simulink model "EPD629_WilliamsJ_AS07_Simulink"  (R2021b)
settings: Solver=VariableStepAuto  StartTime=0.0  StopTime=30  MaxStep=0.01  RelTol=1e-3
values from neighbouring files (symbols this model uses):
  AirGasConstant_kJpkgK = 0.287    [EPD629_WilliamsJ_AS07.m]
  AirToFuelEquivalenceRatio_frac = 1    [EPD629_WilliamsJ_AS07.m]
  AmbientPressure_kPa = 98    [EPD629_WilliamsJ_AS07.m]
  BaseSparkAdvanceData_deg = min(MBTSparkAdvanceData_deg,BorderlineSparkAdvData_deg)    [EPD629_WilliamsJ_AS07.m]
  CrankAngleIVCToTDC_deg = 170    [EPD629_WilliamsJ_AS07.m]
  CylinderAirMassBreakpoints_mg = 0:25:400    [EPD629_WilliamsJ_AS07.m]
  DelayFuelInjectionToIVC_rev = 0.75    [EPD629_WilliamsJ_AS07.m]
  DelayFuelInjectionToIVCEst_rev = 0.75    [EPD629_WilliamsJ_AS07.m]
  DelayIVCToOxygenSensor_rev = 7    [EPD629_WilliamsJ_AS07.m]
  DischargeCoefficient_frac = 0.7    [EPD629_WilliamsJ_AS07.m]
  EngineDisplacement_L = 2.77    [EPD629_WilliamsJ_AS07.m]
  EngineInertia_kgm2 = 0.2    [EPD629_WilliamsJ_AS07.m]
  EngineMotoringFrictionData_Nm = Beta_0 + Beta_2*Omega_e.^2    [EPD629_WilliamsJ_AS07.m]
  EngineSpeedBreakpoints_rpm = 400:200:5000    [EPD629_WilliamsJ_AS07.m]
  FuelControlIntegralGain = 2e-5    (= 2e-05)    [EPD629_WilliamsJ_AS07.m]
  FuelControlProportionalGain = 5e-6    (= 5e-06)    [EPD629_WilliamsJ_AS07.m]
  FuelInjEvapTimeConstant_s = 0.8    [EPD629_WilliamsJ_AS07.m]
  FuelInjEvapTimeConstantEst_s = 0.8    [EPD629_WilliamsJ_AS07.m]
  FuelInjImpactFactor_frac = 0.3    [EPD629_WilliamsJ_AS07.m]
  FuelInjImpactFactorEst_frac = 0.3    [EPD629_WilliamsJ_AS07.m]
  FuelLowerHeatingValue_kJpkg = 44000    [EPD629_WilliamsJ_AS07.m]
  InletAirTemperature_K = 298    [EPD629_WilliamsJ_AS07.m]
  IntakeManifoldVolume_L = 5.8    [EPD629_WilliamsJ_AS07.m]
  ManifoldAirTemperature_K = 340    [EPD629_WilliamsJ_AS07.m]
  ManifoldPressureBreakpoints_kPa = 5:5:100    [EPD629_WilliamsJ_AS07.m]
  NumberOfCylinders = 6    [EPD629_WilliamsJ_AS07.m]
  OxygenSensorLambdaBP_frac = [0 0.9 0.92 0.94 0.96 0.985 0.999 1.001 1.015 1.04 1.06 1.08 1.1 2]    [EPD629_WilliamsJ_AS07.m]
  OxygenSensorSwitchSetpoint_mV = 450    [EPD629_WilliamsJ_AS07.m]
  OxygenSensorVoltageData_mV = [800 800 794 788 775 750 700 200 150 125 112 106 100 100]    [EPD629_WilliamsJ_AS07.m]
  SparkTorqFactorData_frac = 1 - (SparkTorqFactorRetFromMBTBP_deg.^2) /      (SparkTorqFactorRetFromMBTBP_deg(end)^2)    [EPD629_WilliamsJ_AS07.m]
  SparkTorqFactorRetFromMBTBP_deg = 0:5:45    [EPD629_WilliamsJ_AS07.m]
  StoichiometricAFR_frac = 14.7    [EPD629_WilliamsJ_AS07.m]
  ThermodynamicEfficiencyData_frac = Eta_0 + Eta_1*Omega_e + Eta_2*Omega_e.^2    [EPD629_WilliamsJ_AS07.m]
  ThrottleAreaBreakpoints_pct = ThrottleAreaData_pct    [EPD629_WilliamsJ_AS07.m]
  ThrottleAreaData_pct = 100 * ThrottleArea_mm2 / WideOpenThrottleArea_mm2    [EPD629_WilliamsJ_AS07.m]
  ThrottleFlowFunctionData_frac = PR.^(1/RatioOfSpecificHeats_frac) .*      sqrt( 2 * RatioOfSpecificHeats_frac / (RatioOfSpecificHeats_frac - 1) .*      (1 - PR.^((RatioOfSpecificHeats_frac - 1) / RatioOfSpecificHeats_frac)) )    [EPD629_WilliamsJ_AS07.m]
  ThrottleMassFlowCorrIntGain = 10    [EPD629_WilliamsJ_AS07.m]
  ThrottlePositionBreakpoints_pct = 0:100    [EPD629_WilliamsJ_AS07.m]
  ThrottlePositionData_pct = ThrottlePositionBreakpoints_pct    [EPD629_WilliamsJ_AS07.m]
  ThrottlePressureRatioBreakpoints_frac = 0:0.01:1    [EPD629_WilliamsJ_AS07.m]
  VECorrectionFactorIntGain = 0.02    [EPD629_WilliamsJ_AS07.m]
  WideOpenThrottleArea_mm2 = ThrottleArea_mm2(end)    [EPD629_WilliamsJ_AS07.m]
undefined symbols (not defined in the file or in its folder): MBTSparkAdvanceData_deg, VolumetricEfficiencyData_frac
libraries: simulink x1
settings Model: Creator=Justin  LastModifiedBy=jwilli42

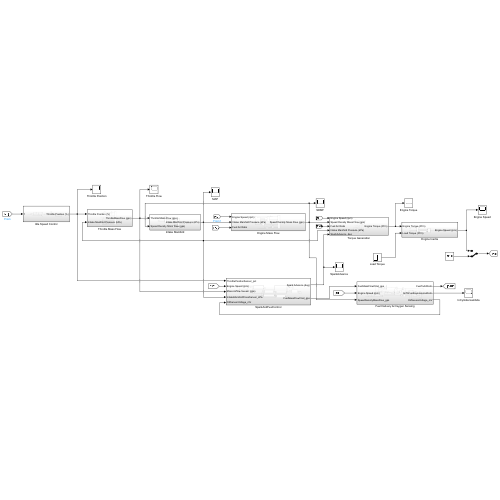
[thumbnail: Simulink's stored preview of the top-level diagram]
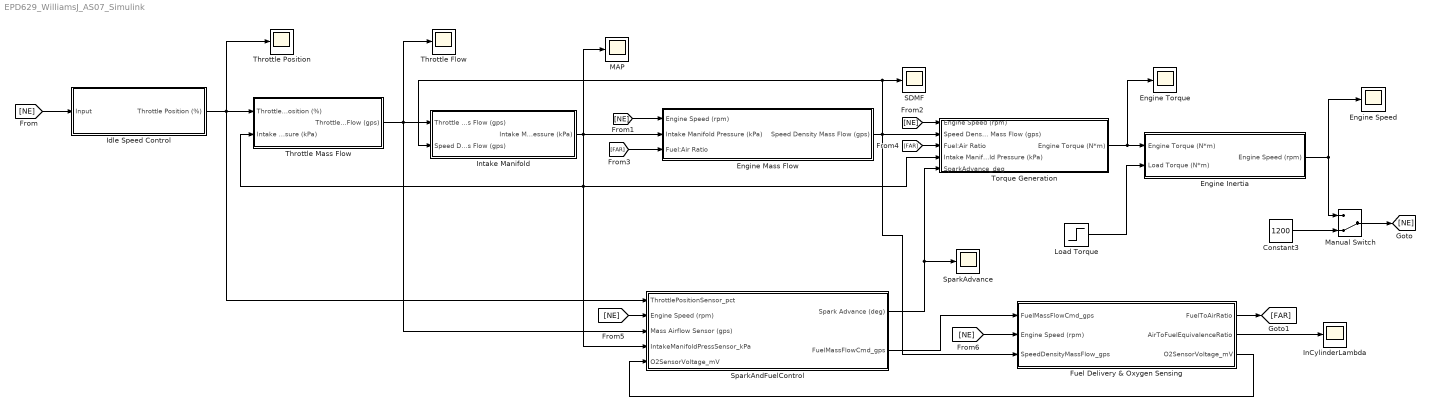
== system EPD629_WilliamsJ_AS07_Simulink ==
  Constant3 : Constant  Value=1200
  Engine Inertia : Subsystem
  Engine Mass Flow : Subsystem
  Engine Speed : Scope
  Engine Torque : Scope
  Fuel Delivery & Oxygen Sensing : Subsystem
  Idle Speed Control : Subsystem
  InCylinderLambda : Scope
  Intake Manifold : Subsystem
  Load Torque : Step  Time=5  Before=15  After=25  SampleTime=0
  MAP : Scope
  Manual Switch : ManualSwitch  CurrentSetting=0
  SDMF : Scope
  SparkAdvance : Scope
  SparkAndFuelControl : Subsystem
  Throttle Flow : Scope
  Throttle Mass Flow : Subsystem
  Throttle Position : Scope
  Torque Generation : Subsystem
  wires:
  Load Torque/1 -> Engine Inertia/2(Load Torque (N*m))
  Idle Speed Control/1(Throttle Position (%)) -> Throttle Mass Flow/1(Throttle Position (%)), SparkAndFuelControl/1(ThrottlePositionSensor_pct), Throttle Position/1
  Intake Manifold/1(Intake Manifold Pressure (kPa)) -> Torque Generation/4(Intake Manifold Pressure (kPa)), SparkAndFuelControl/4(IntakeManifoldPressSensor_kPa), Throttle Mass Flow/2(Intake Manifold Pressure (kPa)), MAP/1, Engine Mass Flow/2(Intake Manifold Pressure (kPa))
  Engine Mass Flow/1(Speed Density Mass Flow (gps)) -> Fuel Delivery & Oxygen Sensing/3(SpeedDensityMassFlow_gps), Torque Generation/2(Speed Density Mass Flow (gps)), SDMF/1, Intake Manifold/2(Speed Density Mass Flow (gps))
  Torque Generation/1(Engine Torque (N*m)) -> Engine Torque/1, Engine Inertia/1(Engine Torque (N*m))
  Engine Inertia/1(Engine Speed (rpm)) -> Engine Speed/1, Manual Switch/1
  [NE] -> Idle Speed Control/1(Input)
  [NE] -> Engine Mass Flow/1(Engine Speed (rpm))
  [NE] -> Torque Generation/1(Engine Speed (rpm))
  [FAR] -> Torque Generation/3(Fuel:Air Ratio)
  [FAR] -> Engine Mass Flow/3(Fuel:Air Ratio)
  Manual Switch/1 -> [NE]
  Constant3/1 -> Manual Switch/2
  SparkAndFuelControl/1(Spark Advance (deg)) -> SparkAdvance/1, Torque Generation/5(SparkAdvance_deg)
  Fuel Delivery & Oxygen Sensing/2(AirToFuelEquivalenceRatio) -> InCylinderLambda/1
  Fuel Delivery & Oxygen Sensing/1(FuelToAirRatio) -> [FAR]
  Fuel Delivery & Oxygen Sensing/3(O2SensorVoltage_mV) -> SparkAndFuelControl/5(O2SensorVoltage_mV)
  [NE] -> SparkAndFuelControl/2(Engine Speed (rpm))
  Throttle Mass Flow/1(ThrottleMassFlow (gps)) -> SparkAndFuelControl/3(Mass Airflow Sensor (gps)), Intake Manifold/1(Throttle Mass Flow (gps)), Throttle Flow/1
  [NE] -> Fuel Delivery & Oxygen Sensing/2(Engine Speed (rpm))
  SparkAndFuelControl/2(FuelMassFlowCmd_gps) -> Fuel Delivery & Oxygen Sensing/1(FuelMassFlowCmd_gps)

== system EPD629_WilliamsJ_AS07_Simulink/Engine Inertia ==
  Engine Torque (N*m) : Inport
  Load Torque (N*m) : Inport  Port=2
  Constant : Constant  Value=EngineInertia_kgm2
  Divide : Product  Inputs=*/
  Engine Speed : Integrator  InitialCondition=600  LimitOutput=on  UpperSaturationLimit=5000  LowerSaturationLimit=0
  Subtract : Sum  Inputs=+-
  rad/s^2 to rpm/s : Gain  Gain=30/pi
  Engine Speed (rpm) : Outport
  wires:
  Engine Torque (N*m)/1 -> Subtract/1
  Load Torque (N*m)/1 -> Subtract/2
  Subtract/1 -> Divide/1
  Constant/1 -> Divide/2
  Divide/1 -> rad/s^2 to rpm/s/1
  rad/s^2 to rpm/s/1 -> Engine Speed/1
  Engine Speed/1 -> Engine Speed (rpm)/1

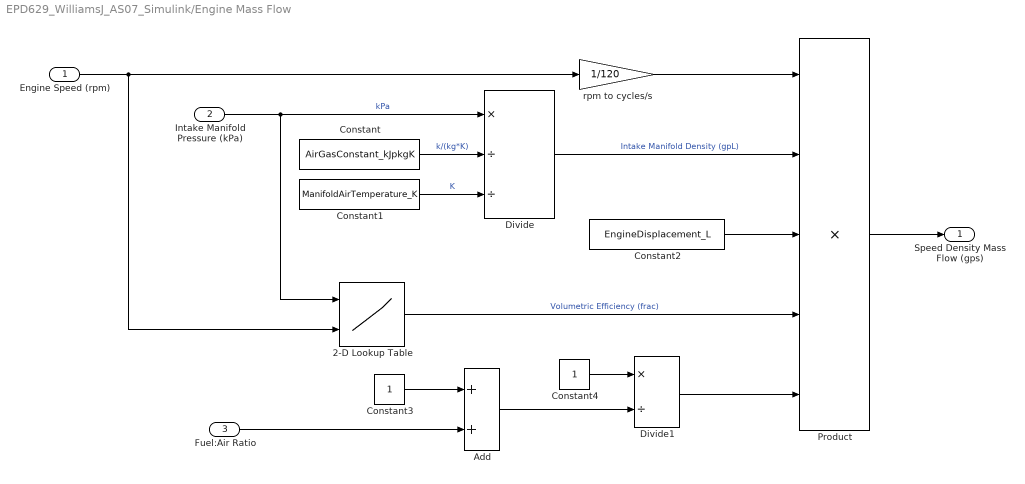
== system EPD629_WilliamsJ_AS07_Simulink/Engine Mass Flow ==
  Engine Speed (rpm) : Inport
  Intake Manifold Pressure (kPa) : Inport  Port=2
  Fuel:Air Ratio : Inport  Port=3
  2-D Lookup Table : Lookup_n-D  BreakpointsForDimension1=ManifoldPressureBreakpoints_kPa  BreakpointsForDimension2=EngineSpeedBreakpoints_rpm  Table=VolumetricEfficiencyData_frac  ExtrapMethod=Clip  UseLastTableValue=on  InternalRulePriority=Speed  RndMeth=Simplest  InputSameDT=on
      settings: InputPortMap=u0,u1
  Add : Sum
  Constant : Constant  Value=AirGasConstant_kJpkgK
  Constant1 : Constant  Value=ManifoldAirTemperature_K
  Constant2 : Constant  Value=EngineDisplacement_L
  Constant3 : Constant
  Constant4 : Constant
  Divide : Product  Inputs=*//
  Divide1 : Product  Inputs=*/
  Product : Product  Inputs=5
  rpm to cycles/s : Gain  Gain=1/120
  Speed Density Mass Flow (gps) : Outport
  wires:
  Engine Speed (rpm)/1 -> rpm to cycles/s/1, 2-D Lookup Table/2
  Intake Manifold Pressure (kPa)/1 -> Divide/1, 2-D Lookup Table/1  "kPa"
  Constant/1 -> Divide/2  "k/(kg*K)"
  Constant1/1 -> Divide/3  "K"
  rpm to cycles/s/1 -> Product/1
  Divide/1 -> Product/2  "Intake Manifold Density (gpL)"
  Constant2/1 -> Product/3
  2-D Lookup Table/1 -> Product/4  "Volumetric Efficiency (frac)"
  Constant3/1 -> Add/1
  Fuel:Air Ratio/1 -> Add/2
  Constant4/1 -> Divide1/1
  Add/1 -> Divide1/2
  Divide1/1 -> Product/5
  Product/1 -> Speed Density Mass Flow (gps)/1

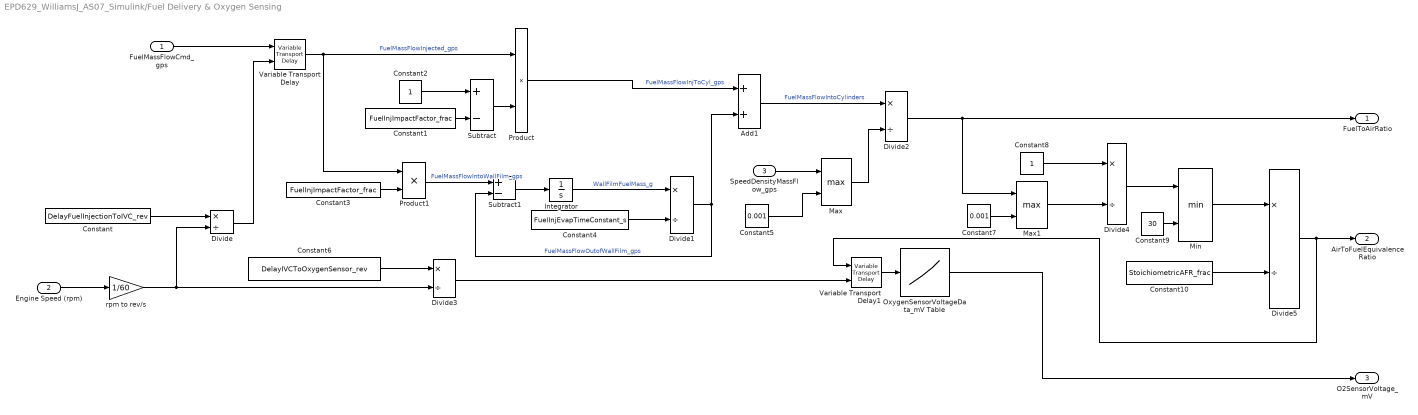
== system EPD629_WilliamsJ_AS07_Simulink/Fuel Delivery & Oxygen Sensing ==
  FuelMassFlowCmd_gps : Inport
  Engine Speed (rpm) : Inport  Port=2
  SpeedDensityMassFlow_gps : Inport  Port=3
  Add1 : Sum
  Constant : Constant  Value=DelayFuelInjectionToIVC_rev
  Constant1 : Constant  Value=FuelInjImpactFactor_frac
  Constant10 : Constant  Value=StoichiometricAFR_frac
  Constant2 : Constant
  Constant3 : Constant  Value=FuelInjImpactFactor_frac
  Constant4 : Constant  Value=FuelInjEvapTimeConstant_s
  Constant5 : Constant  Value=0.001
  Constant6 : Constant  Value=DelayIVCToOxygenSensor_rev
  Constant7 : Constant  Value=0.001
  Constant8 : Constant
  Constant9 : Constant  Value=30
  Divide{,1..5} (6 alike) : Product  Inputs=*/
  Integrator : Integrator  InitialCondition=.015  LimitOutput=on  LowerSaturationLimit=0
  Max : MinMax  Function=max  Inputs=2
  Max1 : MinMax  Function=max  Inputs=2
  Min : MinMax  Inputs=2
  OxygenSensorVoltageData_mV Table : Lookup_n-D  NumberOfTableDimensions=1  BreakpointsForDimension1=OxygenSensorLambdaBP_frac  Table=OxygenSensorVoltageData_mV  ExtrapMethod=Clip  UseLastTableValue=on  InternalRulePriority=Speed  RndMeth=Simplest  InputSameDT=on
  Product : Product
  Product1 : Product
  Subtract : Sum  Inputs=+-
  Subtract1 : Sum  Inputs=+-
  Variable Transport Delay : VariableTransportDelay  VariableDelayType=Variable transport delay  MaximumDelay=10  InitialOutput=.165  MaximumPoints=10000
  Variable Transport Delay1 : VariableTransportDelay  VariableDelayType=Variable transport delay  MaximumDelay=10  InitialOutput=1
  rpm to rev/s : Gain  Gain=1/60
  FuelToAirRatio : Outport
  AirToFuelEquivalenceRatio : Outport  Port=2
  O2SensorVoltage_mV : Outport  Port=3
  wires:
  FuelMassFlowCmd_gps/1 -> Variable Transport Delay/1
  Engine Speed (rpm)/1 -> rpm to rev/s/1
  Constant/1 -> Divide/1
  rpm to rev/s/1 -> Divide/2, Divide3/2
  Divide/1 -> Variable Transport Delay/2
  Constant1/1 -> Subtract/2
  Constant2/1 -> Subtract/1
  Subtract/1 -> Product/2
  Variable Transport Delay/1 -> Product1/1, Product/1  "FuelMassFlowInjected_gps"
  Product/1 -> Add1/1  "FuelMassFlowInjToCyl_gps"
  Constant3/1 -> Product1/2
  Product1/1 -> Subtract1/1  "FuelMassFlowIntoWallFilm_gps"
  Subtract1/1 -> Integrator/1
  Integrator/1 -> Divide1/1  "WallFilmFuelMass_g"
  Constant4/1 -> Divide1/2
  Divide1/1 -> Add1/2, Subtract1/2  "FuelMassFlowOutofWallFilm_gps"
  Add1/1 -> Divide2/1  "FuelMassFlowIntoCylinders"
  SpeedDensityMassFlow_gps/1 -> Max/1
  Constant5/1 -> Max/2
  Max/1 -> Divide2/2
  Constant6/1 -> Divide3/1
  Divide3/1 -> Variable Transport Delay1/2
  Constant7/1 -> Max1/2
  Max1/1 -> Divide4/2
  Constant8/1 -> Divide4/1
  Divide2/1 -> FuelToAirRatio/1, Max1/1
  Divide4/1 -> Min/1
  Constant9/1 -> Min/2
  Constant10/1 -> Divide5/2
  Min/1 -> Divide5/1
  Divide5/1 -> Variable Transport Delay1/1, AirToFuelEquivalenceRatio/1
  Variable Transport Delay1/1 -> OxygenSensorVoltageData_mV Table/1
  OxygenSensorVoltageData_mV Table/1 -> O2SensorVoltage_mV/1

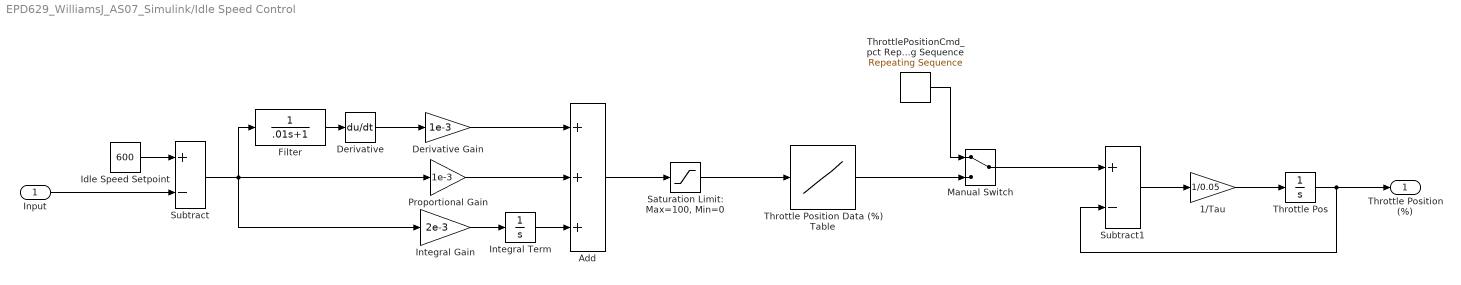
== system EPD629_WilliamsJ_AS07_Simulink/Idle Speed Control ==
  Input : Inport
  1/Tau : Gain  Gain=1/0.05
  Add : Sum  Inputs=+++
  Derivative : Derivative
  Derivative Gain : Gain  Gain=1e-3
  Filter : TransferFcn  Denominator=[.01 1]
  Idle Speed Setpoint : Constant  Value=600
  Integral Gain : Gain  Gain=2e-3
  Integral Term : Integrator  InitialCondition=0.6  LimitOutput=on  UpperSaturationLimit=100  LowerSaturationLimit=0
  Manual Switch : ManualSwitch
  Proportional Gain : Gain  Gain=1e-3
  "Saturation Limit: Max=100, Min=0" : Saturate  UpperLimit=100  LowerLimit=0
  Subtract : Sum  Inputs=+-
  Subtract1 : Sum  Inputs=+-
  Throttle Pos : Integrator  InitialCondition=1.7  LimitOutput=on  UpperSaturationLimit=100  LowerSaturationLimit=0
  Throttle Position Data (%) Table : Lookup_n-D  NumberOfTableDimensions=1  BreakpointsForDimension1=ThrottleAreaBreakpoints_pct  Table=ThrottlePositionData_pct  ExtrapMethod=Clip  UseLastTableValue=on  InternalRulePriority=Speed  RndMeth=Simplest  InputSameDT=on
  ThrottlePositionCmd_pct Repeating Sequence : simulink/Sources/Repeating Sequence  rep_seq_t=[0, 4.5, 5, 9.5, 10]  rep_seq_y=[5, 5, 15, 15, 5]
  Throttle Position (%) : Outport
  wires:
  Idle Speed Setpoint/1 -> Subtract/1
  Filter/1 -> Derivative/1
  Subtract/1 -> Integral Gain/1, Filter/1, Proportional Gain/1
  Derivative/1 -> Derivative Gain/1
  Derivative Gain/1 -> Add/1
  Proportional Gain/1 -> Add/2
  Integral Gain/1 -> Integral Term/1
  Integral Term/1 -> Add/3
  Input/1 -> Subtract/2
  Add/1 -> "Saturation Limit: Max=100, Min=0"/1
  "Saturation Limit: Max=100, Min=0"/1 -> Throttle Position Data (%) Table/1
  Throttle Position Data (%) Table/1 -> Manual Switch/2
  Subtract1/1 -> 1/Tau/1
  1/Tau/1 -> Throttle Pos/1
  Throttle Pos/1 -> Subtract1/2, Throttle Position (%)/1
  Manual Switch/1 -> Subtract1/1
  ThrottlePositionCmd_pct Repeating Sequence/1 -> Manual Switch/1

== system EPD629_WilliamsJ_AS07_Simulink/Intake Manifold ==
  Throttle Mass Flow (gps) : Inport
  Speed Density Mass Flow (gps) : Inport  Port=2
  Constant : Constant  Value=AirGasConstant_kJpkgK
  Constant1 : Constant  Value=ManifoldAirTemperature_K
  Constant2 : Constant  Value=IntakeManifoldVolume_L
  Divide : Product  Inputs=***/
  MAP (kPa) : Integrator  InitialCondition=33.5  LimitOutput=on  UpperSaturationLimit=110  LowerSaturationLimit=10
  Subtract : Sum  Inputs=+-
  Intake Manifold Pressure (kPa) : Outport
  wires:
  Throttle Mass Flow (gps)/1 -> Subtract/1
  Speed Density Mass Flow (gps)/1 -> Subtract/2
  Subtract/1 -> Divide/1  "dm/dt"
  Constant/1 -> Divide/2
  Constant1/1 -> Divide/3
  Constant2/1 -> Divide/4
  Divide/1 -> MAP (kPa)/1  "dP_m/dt"
  MAP (kPa)/1 -> Intake Manifold Pressure (kPa)/1  "P_m"

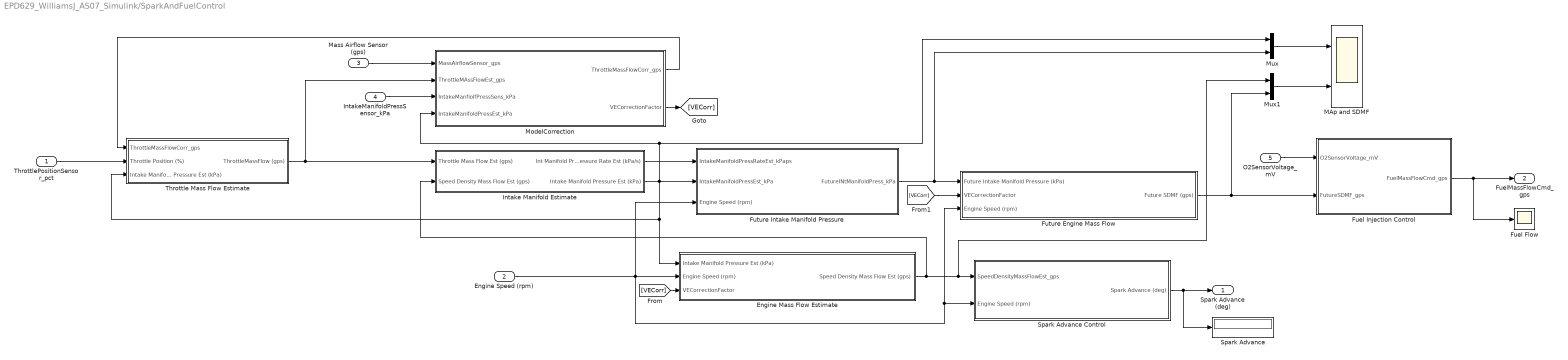
== system EPD629_WilliamsJ_AS07_Simulink/SparkAndFuelControl ==
  ThrottlePositionSensor_pct : Inport
  Engine Speed (rpm) : Inport  Port=2
  Mass Airflow Sensor (gps) : Inport  Port=3
  IntakeManifoldPressSensor_kPa : Inport  Port=4
  O2SensorVoltage_mV : Inport  Port=5
  Engine Mass Flow Estimate : Subsystem
  Fuel Flow : Scope
  "Fuel Injection Control " : Subsystem
  Future Engine Mass Flow : Subsystem
  Future Intake Manifold Pressure : Subsystem
  Intake Manifold Estimate : Subsystem
  MAp and SDMF : Scope  NumInputPorts=2
  ModelCorrection : Subsystem
  Mux : Mux  Inputs=2
  Mux1 : Mux  Inputs=2
  Spark Advance : Display
  Spark Advance Control : Subsystem
  Throttle Mass Flow Estimate : Subsystem
  Spark Advance (deg) : Outport
  FuelMassFlowCmd_gps : Outport  Port=2
  wires:
  Throttle Mass Flow Estimate/1(ThrottleMassFlow (gps)) -> Intake Manifold Estimate/1(Throttle Mass Flow Est (gps)), ModelCorrection/2(ThrottleMAssFlowEst_gps)
  ThrottlePositionSensor_pct/1 -> Throttle Mass Flow Estimate/2(Throttle Position (%))
  ModelCorrection/1(ThrottleMassFlowCorr_gps) -> Throttle Mass Flow Estimate/1(ThrottleMassFlowCorr_gps)
  Engine Speed (rpm)/1 -> Spark Advance Control/2(Engine Speed (rpm)), Future Engine Mass Flow/3(Engine Speed (rpm)), Engine Mass Flow Estimate/2(Engine Speed (rpm)), Future Intake Manifold Pressure/3(Engine Speed (rpm))
  Intake Manifold Estimate/2(Intake Manifold Pressure Est (kPa)) -> Mux/1, ModelCorrection/4(IntakeManifoldPressEst_kPa), Future Intake Manifold Pressure/2(IntakeManifoldPressEst_kPa), Throttle Mass Flow Estimate/3(Intake Manifold Pressure Est (kPa)), Engine Mass Flow Estimate/1(Intake Manifold Pressure Est (kPa))
  Intake Manifold Estimate/1(Int Manifold Pressure Rate Est (kPa/s)) -> Future Intake Manifold Pressure/1(IntakeManifoldPressRateEst_kPaps)
  Engine Mass Flow Estimate/1(Speed Density Mass Flow Est (gps)) -> Intake Manifold Estimate/2(Speed Density Mass Flow Est (gps)), Spark Advance Control/1(SpeedDensityMassFlowEst_gps), Mux1/1
  Future Intake Manifold Pressure/1(FutureINtManifoldPress_kPa) -> Mux/2, Future Engine Mass Flow/1(Future Intake Manifold Pressure (kPa))
  Future Engine Mass Flow/1(Future SDMF (gps)) -> Mux1/2, "Fuel Injection Control "/2(FutureSDMF_gps)
  Spark Advance Control/1(Spark Advance (deg)) -> Spark Advance/1, Spark Advance (deg)/1
  [VECorr] -> Engine Mass Flow Estimate/3(VECorrectionFactor)
  ModelCorrection/2(VECorrectionFactor) -> [VECorr]
  Mass Airflow Sensor (gps)/1 -> ModelCorrection/1(MassAirflowSensor_gps)
  IntakeManifoldPressSensor_kPa/1 -> ModelCorrection/3(IntakeManfiolfPressSens_kPa)
  O2SensorVoltage_mV/1 -> "Fuel Injection Control "/1(O2SensorVoltage_mV)
  "Fuel Injection Control "/1(FuelMassFlowCmd_gps) -> Fuel Flow/1, FuelMassFlowCmd_gps/1
  [VECorr] -> Future Engine Mass Flow/2(VECorrectionFactor)
  Mux/1 -> MAp and SDMF/1
  Mux1/1 -> MAp and SDMF/2

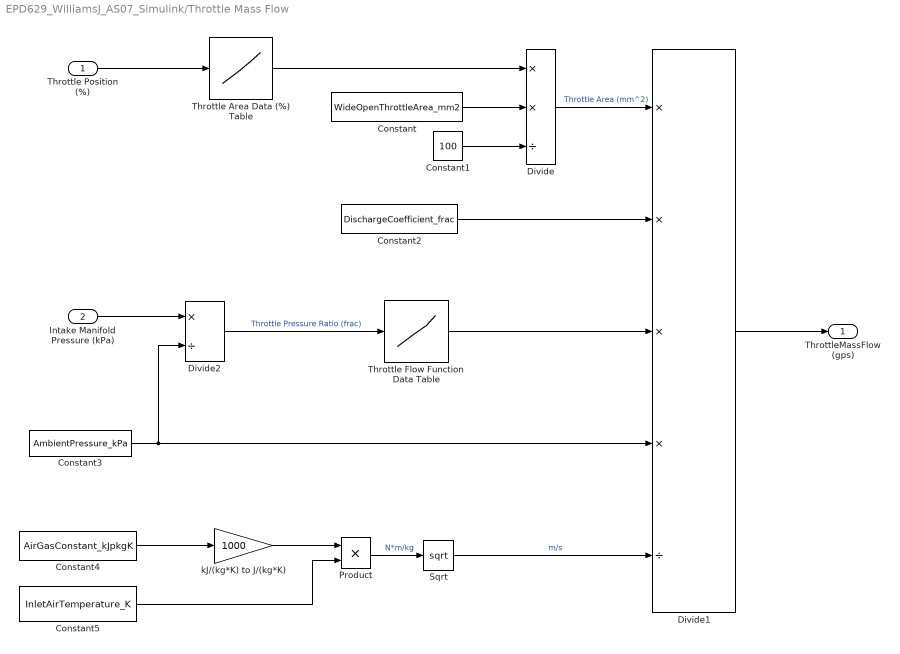
== system EPD629_WilliamsJ_AS07_Simulink/Throttle Mass Flow ==
  Throttle Position (%) : Inport
  Intake Manifold Pressure (kPa) : Inport  Port=2
  Constant : Constant  Value=WideOpenThrottleArea_mm2
  Constant1 : Constant  Value=100
  Constant2 : Constant  Value=DischargeCoefficient_frac
  Constant3 : Constant  Value=AmbientPressure_kPa
  Constant4 : Constant  Value=AirGasConstant_kJpkgK
  Constant5 : Constant  Value=InletAirTemperature_K
  Divide : Product  Inputs=**/
  Divide1 : Product  Inputs=****/
  Divide2 : Product  Inputs=*/
  Product : Product
  Sqrt : Sqrt  SaturateOnIntegerOverflow=on
  Throttle Area Data (%) Table : Lookup_n-D  NumberOfTableDimensions=1  BreakpointsForDimension1=ThrottlePositionBreakpoints_pct  Table=ThrottleAreaData_pct  ExtrapMethod=Clip  UseLastTableValue=on  InternalRulePriority=Speed  RndMeth=Simplest  InputSameDT=on
  Throttle Flow Function Data Table : Lookup_n-D  NumberOfTableDimensions=1  BreakpointsForDimension1=ThrottlePressureRatioBreakpoints_frac  Table=ThrottleFlowFunctionData_frac  ExtrapMethod=Clip  UseLastTableValue=on  InternalRulePriority=Speed  RndMeth=Simplest  InputSameDT=on
  kJ/(kg*K) to J/(kg*K) : Gain  Gain=1000
  ThrottleMassFlow (gps) : Outport
  wires:
  Throttle Position (%)/1 -> Throttle Area Data (%) Table/1
  Throttle Area Data (%) Table/1 -> Divide/1
  Constant/1 -> Divide/2
  Constant1/1 -> Divide/3
  Divide/1 -> Divide1/1  "Throttle Area (mm^2)"
  Constant2/1 -> Divide1/2
  Intake Manifold Pressure (kPa)/1 -> Divide2/1
  Constant3/1 -> Divide2/2, Divide1/4
  Throttle Flow Function Data Table/1 -> Divide1/3
  Divide2/1 -> Throttle Flow Function Data Table/1  "Throttle Pressure Ratio (frac)"
  Constant4/1 -> kJ/(kg*K) to J/(kg*K)/1
  kJ/(kg*K) to J/(kg*K)/1 -> Product/1
  Constant5/1 -> Product/2
  Product/1 -> Sqrt/1  "N*m/kg"
  Sqrt/1 -> Divide1/5  "m/s"
  Divide1/1 -> ThrottleMassFlow (gps)/1

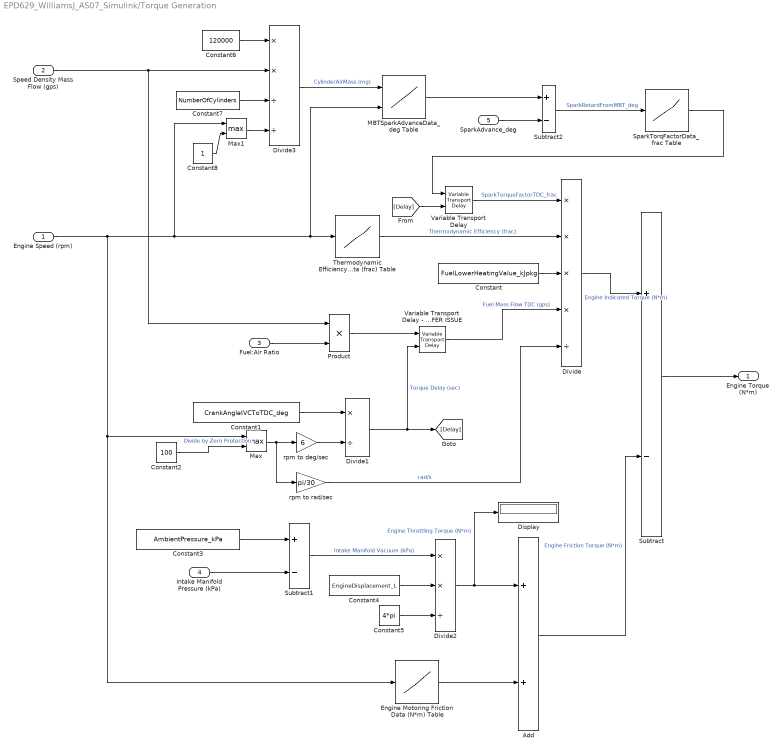
== system EPD629_WilliamsJ_AS07_Simulink/Torque Generation ==
  Engine Speed (rpm) : Inport
  Speed Density Mass Flow (gps) : Inport  Port=2
  Fuel:Air Ratio : Inport  Port=3
  Intake Manifold Pressure (kPa) : Inport  Port=4
  SparkAdvance_deg : Inport  Port=5
  Add : Sum
  Constant : Constant  Value=FuelLowerHeatingValue_kJpkg
  Constant1 : Constant  Value=CrankAngleIVCToTDC_deg
  Constant2 : Constant  Value=100
  Constant3 : Constant  Value=AmbientPressure_kPa
  Constant4 : Constant  Value=EngineDisplacement_L
  Constant5 : Constant  Value=4*pi
  Constant6 : Constant  Value=120000
  Constant7 : Constant  Value=NumberOfCylinders
  Constant8 : Constant
  Display : Display
  Divide : Product  Inputs=****/
  Divide1 : Product  Inputs=*/
  Divide2 : Product  Inputs=**/
  Divide3 : Product  Inputs=**//
  Engine Motoring Friction Data (N*m) Table : Lookup_n-D  NumberOfTableDimensions=1  BreakpointsForDimension1=EngineSpeedBreakpoints_rpm  Table=EngineMotoringFrictionData_Nm  ExtrapMethod=Clip  UseLastTableValue=on  InternalRulePriority=Speed  RndMeth=Simplest  InputSameDT=on
  MBTSparkAdvanceData_deg Table : Lookup_n-D  BreakpointsForDimension1=CylinderAirMassBreakpoints_mg  BreakpointsForDimension2=EngineSpeedBreakpoints_rpm  Table=MBTSparkAdvanceData_deg  ExtrapMethod=Clip  UseLastTableValue=on  InternalRulePriority=Speed  RndMeth=Simplest  InputSameDT=on
      settings: InputPortMap=u0,u1
  Max : MinMax  Function=max  Inputs=2
  Max1 : MinMax  Function=max  Inputs=2
  Product : Product
  SparkTorqFactorData_frac Table : Lookup_n-D  NumberOfTableDimensions=1  BreakpointsForDimension1=SparkTorqFactorRetFromMBTBP_deg  Table=SparkTorqFactorData_frac  ExtrapMethod=Clip  UseLastTableValue=on  InternalRulePriority=Speed  RndMeth=Simplest  InputSameDT=on
  Subtract : Sum  Inputs=+-
  Subtract1 : Sum  Inputs=+-
  Subtract2 : Sum  Inputs=+-
  Thermodynamic Efficiency Data (frac) Table : Lookup_n-D  NumberOfTableDimensions=1  BreakpointsForDimension1=EngineSpeedBreakpoints_rpm  Table=ThermodynamicEfficiencyData_frac  ExtrapMethod=Clip  UseLastTableValue=on  InternalRulePriority=Speed  RndMeth=Simplest  InputSameDT=on
  Variable Transport Delay : VariableTransportDelay  VariableDelayType=Variable transport delay  MaximumDelay=10  InitialOutput=1
  "Variable Transport Delay - BUFFER ISSUE " : VariableTransportDelay  VariableDelayType=Variable transport delay  MaximumDelay=10  InitialOutput=0.166
  rpm to deg/sec : Gain  Gain=6
  rpm to rad/sec : Gain  Gain=pi/30
  Engine Torque (N*m) : Outport
  wires:
  Engine Speed (rpm)/1 -> Engine Motoring Friction Data (N*m) Table/1, Max/1, Max1/1, MBTSparkAdvanceData_deg Table/2, Thermodynamic Efficiency Data (frac) Table/1
  Thermodynamic Efficiency Data (frac) Table/1 -> Divide/2  "Thermodynamic Efficiency (frac)"
  Constant/1 -> Divide/3
  Speed Density Mass Flow (gps)/1 -> Divide3/2, Product/1
  Fuel:Air Ratio/1 -> Product/2
  Product/1 -> "Variable Transport Delay - BUFFER ISSUE "/1
  "Variable Transport Delay - BUFFER ISSUE "/1 -> Divide/4  "Fuel Mass Flow TDC (gps)"
  Constant1/1 -> Divide1/1
  Constant2/1 -> Max/2  "Divide by Zero Protection"
  Max/1 -> rpm to rad/sec/1, rpm to deg/sec/1
  rpm to deg/sec/1 -> Divide1/2
  Divide1/1 -> [Delay], "Variable Transport Delay - BUFFER ISSUE "/2  "Torque Delay (sec)"
  rpm to rad/sec/1 -> Divide/5  "rad/s"
  Divide/1 -> Subtract/1  "Engine Indicated Torque (N*m)"
  Constant3/1 -> Subtract1/1
  Intake Manifold Pressure (kPa)/1 -> Subtract1/2
  Subtract1/1 -> Divide2/1  "Intake Manifold Vacuum (kPa)"
  Constant4/1 -> Divide2/2
  Constant5/1 -> Divide2/3
  Engine Motoring Friction Data (N*m) Table/1 -> Add/2
  Divide2/1 -> Display/1, Add/1  "Engine Throttling Torque (N*m)"
  Add/1 -> Subtract/2  "Engine Friction Torque (N*m)"
  Subtract/1 -> Engine Torque (N*m)/1
  Constant6/1 -> Divide3/1
  Constant7/1 -> Divide3/3
  Max1/1 -> Divide3/4
  Constant8/1 -> Max1/2
  Divide3/1 -> MBTSparkAdvanceData_deg Table/1  "CylinderAirMass (mg)"
  [Delay] -> Variable Transport Delay/2
  Variable Transport Delay/1 -> Divide/1  "SparkTorqueFactorTDC_frac"
  MBTSparkAdvanceData_deg Table/1 -> Subtract2/1
  SparkAdvance_deg/1 -> Subtract2/2
  Subtract2/1 -> SparkTorqFactorData_frac Table/1  "SparkRetardFromMBT_deg"
  SparkTorqFactorData_frac Table/1 -> Variable Transport Delay/1

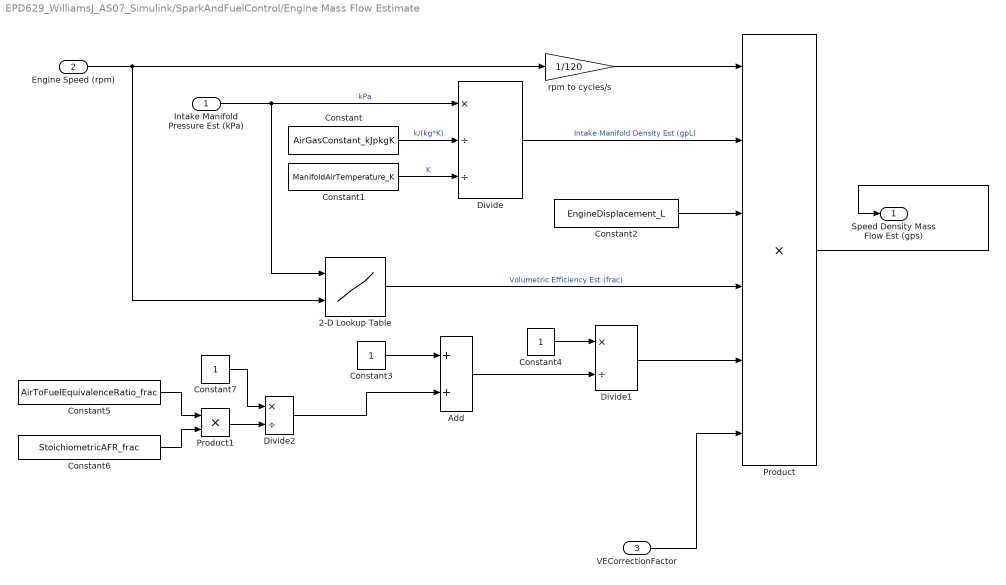
== system EPD629_WilliamsJ_AS07_Simulink/SparkAndFuelControl/Engine Mass Flow Estimate ==
  Intake Manifold Pressure Est (kPa) : Inport
  Engine Speed (rpm) : Inport  Port=2
  VECorrectionFactor : Inport  Port=3
  2-D Lookup Table : Lookup_n-D  BreakpointsForDimension1=ManifoldPressureBreakpoints_kPa  BreakpointsForDimension2=EngineSpeedBreakpoints_rpm  Table=VolumetricEfficiencyData_frac  ExtrapMethod=Clip  UseLastTableValue=on  InternalRulePriority=Speed  RndMeth=Simplest  InputSameDT=on
      settings: InputPortMap=u0,u1
  Add : Sum
  Constant : Constant  Value=AirGasConstant_kJpkgK
  Constant1 : Constant  Value=ManifoldAirTemperature_K
  Constant2 : Constant  Value=EngineDisplacement_L
  Constant3 : Constant
  Constant4 : Constant
  Constant5 : Constant  Value=AirToFuelEquivalenceRatio_frac
  Constant6 : Constant  Value=StoichiometricAFR_frac
  Constant7 : Constant
  Divide : Product  Inputs=*//
  Divide1 : Product  Inputs=*/
  Divide2 : Product  Inputs=*/
  Product : Product  Inputs=6
  Product1 : Product
  rpm to cycles/s : Gain  Gain=1/120
  Speed Density Mass Flow Est (gps) : Outport
  wires:
  Engine Speed (rpm)/1 -> rpm to cycles/s/1, 2-D Lookup Table/2
  Intake Manifold Pressure Est (kPa)/1 -> Divide/1, 2-D Lookup Table/1  "kPa"
  Constant/1 -> Divide/2  "k/(kg*K)"
  Constant1/1 -> Divide/3  "K"
  rpm to cycles/s/1 -> Product/1
  Divide/1 -> Product/2  "Intake Manifold Density Est (gpL)"
  Constant2/1 -> Product/3
  2-D Lookup Table/1 -> Product/4  "Volumetric Efficiency Est (frac)"
  Constant3/1 -> Add/1
  Constant4/1 -> Divide1/1
  Add/1 -> Divide1/2
  Divide1/1 -> Product/5
  Product/1 -> Speed Density Mass Flow Est (gps)/1
  VECorrectionFactor/1 -> Product/6
  Constant6/1 -> Product1/2
  Constant5/1 -> Product1/1
  Product1/1 -> Divide2/2
  Constant7/1 -> Divide2/1
  Divide2/1 -> Add/2

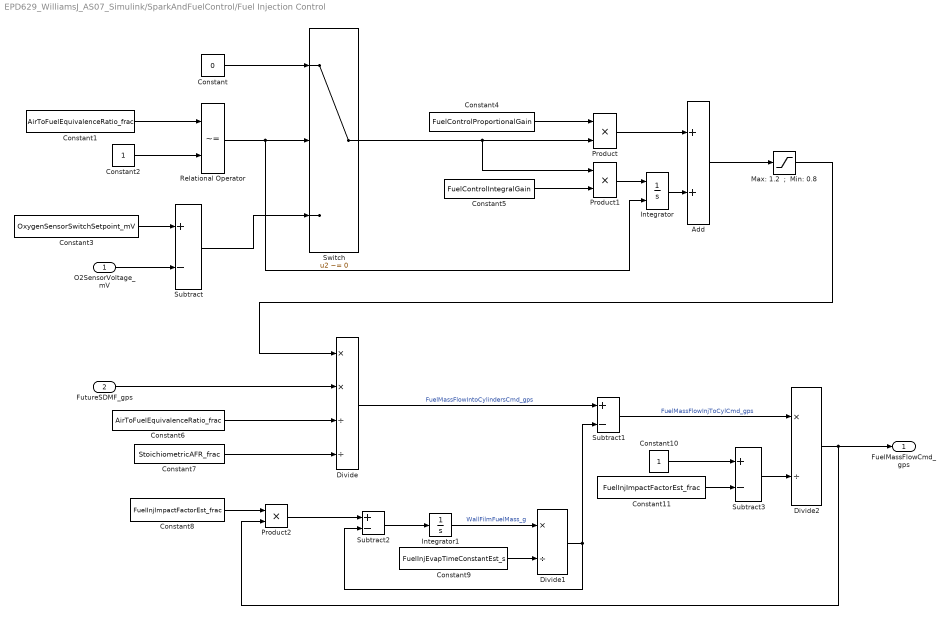
== system EPD629_WilliamsJ_AS07_Simulink/SparkAndFuelControl/Fuel Injection Control  ==
  O2SensorVoltage_mV : Inport
  FutureSDMF_gps : Inport  Port=2
  Add : Sum
  Constant : Constant  Value=0
  Constant1 : Constant  Value=AirToFuelEquivalenceRatio_frac
  Constant10 : Constant
  Constant11 : Constant  Value=FuelInjImpactFactorEst_frac
  Constant2 : Constant
  Constant3 : Constant  Value=OxygenSensorSwitchSetpoint_mV
  Constant4 : Constant  Value=FuelControlProportionalGain
  Constant5 : Constant  Value=FuelControlIntegralGain
  Constant6 : Constant  Value=AirToFuelEquivalenceRatio_frac
  Constant7 : Constant  Value=StoichiometricAFR_frac
  Constant8 : Constant  Value=FuelInjImpactFactorEst_frac
  Constant9 : Constant  Value=FuelInjEvapTimeConstantEst_s
  Divide : Product  Inputs=**//
  Divide1 : Product  Inputs=*/
  Divide2 : Product  Inputs=*/
  Integrator : Integrator  ExternalReset=level hold  InitialCondition=1  LimitOutput=on  UpperSaturationLimit=1.2  LowerSaturationLimit=0.8
  Integrator1 : Integrator  InitialCondition=0.015  LimitOutput=on  LowerSaturationLimit=0
  Max: 1.2  ;  Min: 0.8 : Saturate  UpperLimit=1.2  LowerLimit=0.8
  Product : Product
  Product1 : Product
  Product2 : Product
  Relational Operator : RelationalOperator  Operator=~=  OutDataTypeStr=boolean  RndMeth=Simplest
  Subtract{,1..3} (4 alike) : Sum  Inputs=+-
  Switch : Switch  Criteria=u2 ~= 0
  FuelMassFlowCmd_gps : Outport
  wires:
  Constant/1 -> Switch/1
  Constant3/1 -> Subtract/1
  O2SensorVoltage_mV/1 -> Subtract/2
  Constant1/1 -> Relational Operator/1
  Constant2/1 -> Relational Operator/2
  Relational Operator/1 -> Integrator/2, Switch/2
  Subtract/1 -> Switch/3
  Switch/1 -> Product1/1, Product/2
  Constant4/1 -> Product/1
  Constant5/1 -> Product1/2
  Product1/1 -> Integrator/1
  Product/1 -> Add/1
  Integrator/1 -> Add/2
  Add/1 -> Max: 1.2  ;  Min: 0.8/1
  Max: 1.2  ;  Min: 0.8/1 -> Divide/1
  FutureSDMF_gps/1 -> Divide/2
  Constant6/1 -> Divide/3
  Constant7/1 -> Divide/4
  Divide/1 -> Subtract1/1  "FuelMassFlowIntoCylindersCmd_gps"
  Product2/1 -> Subtract2/1
  Subtract2/1 -> Integrator1/1
  Integrator1/1 -> Divide1/1  "WallFilmFuelMass_g"
  Constant8/1 -> Product2/1
  Constant9/1 -> Divide1/2
  Divide1/1 -> Subtract2/2, Subtract1/2
  Subtract1/1 -> Divide2/1  "FuelMassFlowInjToCylCmd_gps"
  Constant10/1 -> Subtract3/1
  Constant11/1 -> Subtract3/2
  Subtract3/1 -> Divide2/2
  Divide2/1 -> FuelMassFlowCmd_gps/1, Product2/2

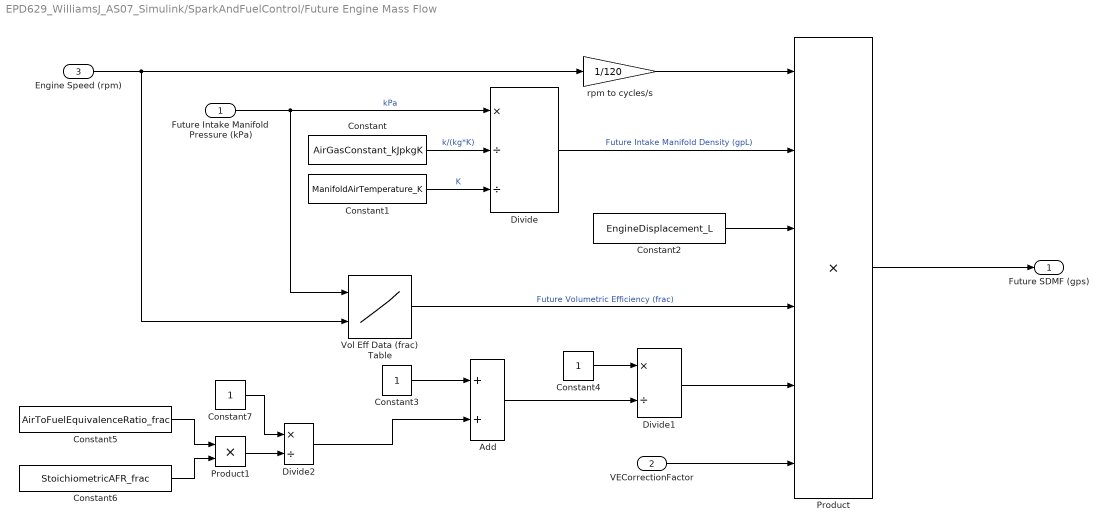
== system EPD629_WilliamsJ_AS07_Simulink/SparkAndFuelControl/Future Engine Mass Flow ==
  Future Intake Manifold Pressure (kPa) : Inport
  VECorrectionFactor : Inport  Port=2
  Engine Speed (rpm) : Inport  Port=3
  Add : Sum
  Constant : Constant  Value=AirGasConstant_kJpkgK
  Constant1 : Constant  Value=ManifoldAirTemperature_K
  Constant2 : Constant  Value=EngineDisplacement_L
  Constant3 : Constant
  Constant4 : Constant
  Constant5 : Constant  Value=AirToFuelEquivalenceRatio_frac
  Constant6 : Constant  Value=StoichiometricAFR_frac
  Constant7 : Constant
  Divide : Product  Inputs=*//
  Divide1 : Product  Inputs=*/
  Divide2 : Product  Inputs=*/
  Product : Product  Inputs=6
  Product1 : Product
  Vol Eff Data (frac) Table : Lookup_n-D  BreakpointsForDimension1=ManifoldPressureBreakpoints_kPa  BreakpointsForDimension2=EngineSpeedBreakpoints_rpm  Table=VolumetricEfficiencyData_frac  ExtrapMethod=Clip  UseLastTableValue=on  InternalRulePriority=Speed  RndMeth=Simplest  InputSameDT=on
      settings: InputPortMap=u0,u1
  rpm to cycles/s : Gain  Gain=1/120
  Future SDMF (gps) : Outport
  wires:
  Engine Speed (rpm)/1 -> rpm to cycles/s/1, Vol Eff Data (frac) Table/2
  Future Intake Manifold Pressure (kPa)/1 -> Divide/1, Vol Eff Data (frac) Table/1  "kPa"
  Constant/1 -> Divide/2  "k/(kg*K)"
  Constant1/1 -> Divide/3  "K"
  rpm to cycles/s/1 -> Product/1
  Divide/1 -> Product/2  "Future Intake Manifold Density (gpL)"
  Constant2/1 -> Product/3
  Vol Eff Data (frac) Table/1 -> Product/4  "Future Volumetric Efficiency (frac)"
  Constant3/1 -> Add/1
  Constant4/1 -> Divide1/1
  Add/1 -> Divide1/2
  Divide1/1 -> Product/5
  Product/1 -> Future SDMF (gps)/1
  VECorrectionFactor/1 -> Product/6
  Constant6/1 -> Product1/2
  Constant5/1 -> Product1/1
  Product1/1 -> Divide2/2
  Constant7/1 -> Divide2/1
  Divide2/1 -> Add/2

== system EPD629_WilliamsJ_AS07_Simulink/SparkAndFuelControl/Future Intake Manifold Pressure ==
  IntakeManifoldPressRateEst_kPaps : Inport
  IntakeManifoldPressEst_kPa : Inport  Port=2
  Engine Speed (rpm) : Inport  Port=3
  Add : Sum
  Constant : Constant  Value=DelayFuelInjectionToIVCEst_rev
  Divide : Product  Inputs=*/
  Product : Product
  rpm to rev/s : Gain  Gain=1/60
  FutureINtManifoldPress_kPa : Outport
  wires:
  Engine Speed (rpm)/1 -> rpm to rev/s/1
  Constant/1 -> Divide/1
  rpm to rev/s/1 -> Divide/2
  Divide/1 -> Product/2
  IntakeManifoldPressRateEst_kPaps/1 -> Product/1
  Product/1 -> Add/2  "FutureDeltaIntManPress_kPa"
  IntakeManifoldPressEst_kPa/1 -> Add/1
  Add/1 -> FutureINtManifoldPress_kPa/1

== system EPD629_WilliamsJ_AS07_Simulink/SparkAndFuelControl/Intake Manifold Estimate ==
  Throttle Mass Flow Est (gps) : Inport
  Speed Density Mass Flow Est (gps) : Inport  Port=2
  Constant : Constant  Value=AirGasConstant_kJpkgK
  Constant1 : Constant  Value=ManifoldAirTemperature_K
  Constant2 : Constant  Value=IntakeManifoldVolume_L
  Divide : Product  Inputs=***/
  MAP (kPa) : Integrator  InitialCondition=33.5  LimitOutput=on  UpperSaturationLimit=110  LowerSaturationLimit=10
  Subtract : Sum  Inputs=+-
  Int Manifold Pressure Rate Est (kPa/s) : Outport
  Intake Manifold Pressure Est (kPa) : Outport  Port=2
  wires:
  Throttle Mass Flow Est (gps)/1 -> Subtract/1
  Speed Density Mass Flow Est (gps)/1 -> Subtract/2
  Subtract/1 -> Divide/1  "dm/dt"
  Constant/1 -> Divide/2
  Constant1/1 -> Divide/3
  Constant2/1 -> Divide/4
  Divide/1 -> MAP (kPa)/1, Int Manifold Pressure Rate Est (kPa/s)/1  "dP_m/dt"
  MAP (kPa)/1 -> Intake Manifold Pressure Est (kPa)/1  "P_m"

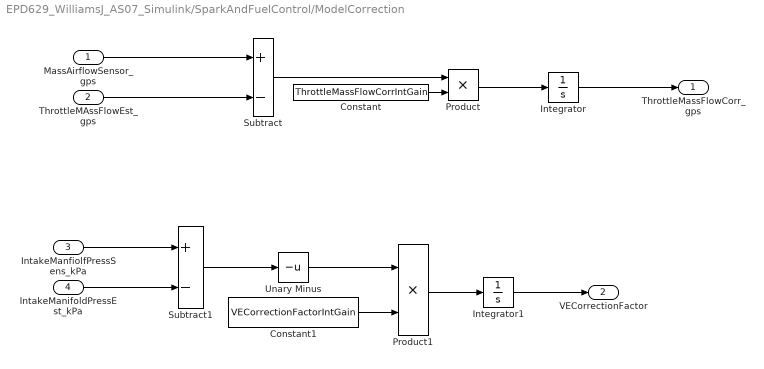
== system EPD629_WilliamsJ_AS07_Simulink/SparkAndFuelControl/ModelCorrection ==
  MassAirflowSensor_gps : Inport
  ThrottleMAssFlowEst_gps : Inport  Port=2
  IntakeManfiolfPressSens_kPa : Inport  Port=3
  IntakeManifoldPressEst_kPa : Inport  Port=4
  Constant : Constant  Value=ThrottleMassFlowCorrIntGain
  Constant1 : Constant  Value=VECorrectionFactorIntGain
  Integrator : Integrator  LimitOutput=on  UpperSaturationLimit=100  LowerSaturationLimit=-100
  Integrator1 : Integrator  InitialCondition=1  LimitOutput=on  UpperSaturationLimit=2  LowerSaturationLimit=0.5
  Product : Product
  Product1 : Product
  Subtract : Sum  Inputs=+-
  Subtract1 : Sum  Inputs=+-
  Unary Minus : UnaryMinus
  ThrottleMassFlowCorr_gps : Outport
  VECorrectionFactor : Outport  Port=2
  wires:
  MassAirflowSensor_gps/1 -> Subtract/1
  ThrottleMAssFlowEst_gps/1 -> Subtract/2
  Subtract/1 -> Product/1
  Constant/1 -> Product/2
  Integrator/1 -> ThrottleMassFlowCorr_gps/1
  Product/1 -> Integrator/1
  IntakeManfiolfPressSens_kPa/1 -> Subtract1/1
  IntakeManifoldPressEst_kPa/1 -> Subtract1/2
  Subtract1/1 -> Unary Minus/1
  Unary Minus/1 -> Product1/1
  Constant1/1 -> Product1/2
  Product1/1 -> Integrator1/1
  Integrator1/1 -> VECorrectionFactor/1

== system EPD629_WilliamsJ_AS07_Simulink/SparkAndFuelControl/Spark Advance Control ==
  SpeedDensityMassFlowEst_gps : Inport
  Engine Speed (rpm) : Inport  Port=2
  Base Spark Advance Data (deg) Table : Lookup_n-D  BreakpointsForDimension1=CylinderAirMassBreakpoints_mg  BreakpointsForDimension2=EngineSpeedBreakpoints_rpm  Table=BaseSparkAdvanceData_deg  ExtrapMethod=Clip  UseLastTableValue=on  InternalRulePriority=Speed  RndMeth=Simplest  InputSameDT=on
      settings: InputPortMap=u0,u1
  Constant : Constant  Value=120000
  Constant1 : Constant  Value=NumberOfCylinders
  Constant2 : Constant
  Divide : Product  Inputs=**//
  Max : MinMax  Function=max  Inputs=2
  Spark Advance (deg) : Outport
  wires:
  SpeedDensityMassFlowEst_gps/1 -> Divide/2
  Constant/1 -> Divide/1
  Constant1/1 -> Divide/3
  Constant2/1 -> Max/2
  Engine Speed (rpm)/1 -> Base Spark Advance Data (deg) Table/2, Max/1
  Max/1 -> Divide/4
  Divide/1 -> Base Spark Advance Data (deg) Table/1
  Base Spark Advance Data (deg) Table/1 -> Spark Advance (deg)/1

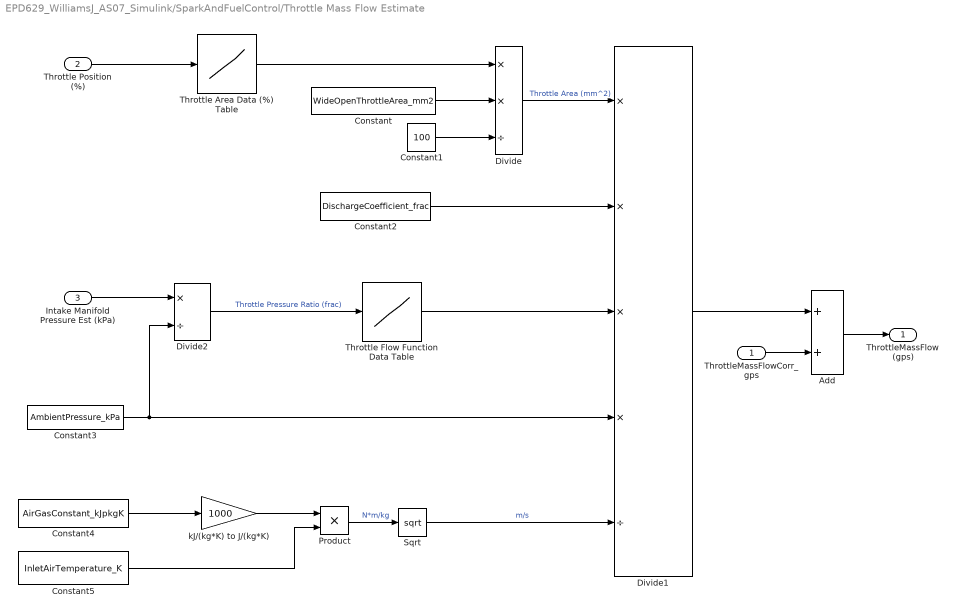
== system EPD629_WilliamsJ_AS07_Simulink/SparkAndFuelControl/Throttle Mass Flow Estimate ==
  ThrottleMassFlowCorr_gps : Inport
  Throttle Position (%) : Inport  Port=2
  Intake Manifold Pressure Est (kPa) : Inport  Port=3
  Add : Sum
  Constant : Constant  Value=WideOpenThrottleArea_mm2
  Constant1 : Constant  Value=100
  Constant2 : Constant  Value=DischargeCoefficient_frac
  Constant3 : Constant  Value=AmbientPressure_kPa
  Constant4 : Constant  Value=AirGasConstant_kJpkgK
  Constant5 : Constant  Value=InletAirTemperature_K
  Divide : Product  Inputs=**/
  Divide1 : Product  Inputs=****/
  Divide2 : Product  Inputs=*/
  Product : Product
  Sqrt : Sqrt  SaturateOnIntegerOverflow=on
  Throttle Area Data (%) Table : Lookup_n-D  NumberOfTableDimensions=1  BreakpointsForDimension1=ThrottlePositionBreakpoints_pct  Table=ThrottleAreaData_pct  ExtrapMethod=Clip  UseLastTableValue=on  InternalRulePriority=Speed  RndMeth=Simplest  InputSameDT=on
  Throttle Flow Function Data Table : Lookup_n-D  NumberOfTableDimensions=1  BreakpointsForDimension1=ThrottlePressureRatioBreakpoints_frac  Table=ThrottleFlowFunctionData_frac  ExtrapMethod=Clip  UseLastTableValue=on  InternalRulePriority=Speed  RndMeth=Simplest  InputSameDT=on
  kJ/(kg*K) to J/(kg*K) : Gain  Gain=1000
  ThrottleMassFlow (gps) : Outport
  wires:
  Throttle Position (%)/1 -> Throttle Area Data (%) Table/1
  Throttle Area Data (%) Table/1 -> Divide/1
  Constant/1 -> Divide/2
  Constant1/1 -> Divide/3
  Divide/1 -> Divide1/1  "Throttle Area (mm^2)"
  Constant2/1 -> Divide1/2
  Intake Manifold Pressure Est (kPa)/1 -> Divide2/1
  Constant3/1 -> Divide2/2, Divide1/4
  Throttle Flow Function Data Table/1 -> Divide1/3
  Divide2/1 -> Throttle Flow Function Data Table/1  "Throttle Pressure Ratio (frac)"
  Constant4/1 -> kJ/(kg*K) to J/(kg*K)/1
  kJ/(kg*K) to J/(kg*K)/1 -> Product/1
  Constant5/1 -> Product/2
  Product/1 -> Sqrt/1  "N*m/kg"
  Sqrt/1 -> Divide1/5  "m/s"
  Add/1 -> ThrottleMassFlow (gps)/1
  Divide1/1 -> Add/1
  ThrottleMassFlowCorr_gps/1 -> Add/2
